simulink model "TorqueSnake"  (R2015b)
settings: Solver=FixedStepAuto  StartTime=0.0  StopTime=tmax  FixedStep=0.01  RelTol=1e-3
values from neighbouring files (symbols this model uses):
  c1 = 0.45    [PreSim.m]
  c2 = 3    [PreSim.m]
  Ms = 1    [PreSim.m]
  N = 3    [PreSim.m]
settings Model: Creator=Christian Dos Santos  LastModifiedBy=Christian Dos Santos

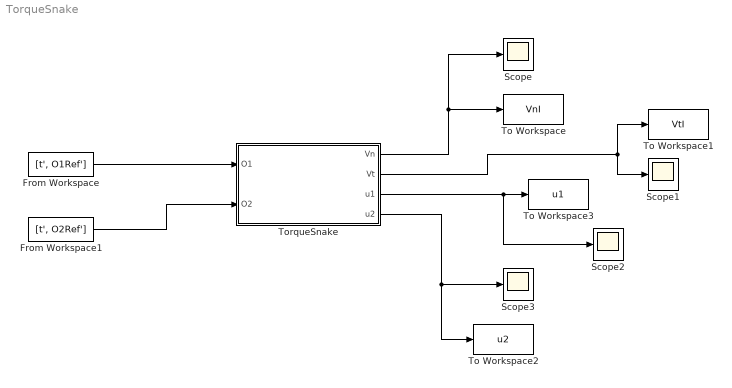
== system TorqueSnake ==
  From Workspace : FromWorkspace  VariableName=[t', O1Ref']
  From Workspace1 : FromWorkspace  VariableName=[t', O2Ref']
  Scope{,1..3} (4 alike) : Scope
  To Workspace : ToWorkspace  VariableName=VnI  SampleTime=-1
  To Workspace1 : ToWorkspace  VariableName=VtI  SampleTime=-1
  To Workspace2 : ToWorkspace  VariableName=u2  SampleTime=-1
  To Workspace3 : ToWorkspace  VariableName=u1  SampleTime=-1
  TorqueSnake : Subsystem
  wires:
  From Workspace/1 -> TorqueSnake/1(O1)
  From Workspace1/1 -> TorqueSnake/2(O2)
  TorqueSnake/1(Vn) -> To Workspace/1, Scope/1
  TorqueSnake/2("Vt ") -> Scope1/1, To Workspace1/1
  TorqueSnake/3(u1) -> To Workspace3/1, Scope2/1
  TorqueSnake/4(u2) -> To Workspace2/1, Scope3/1

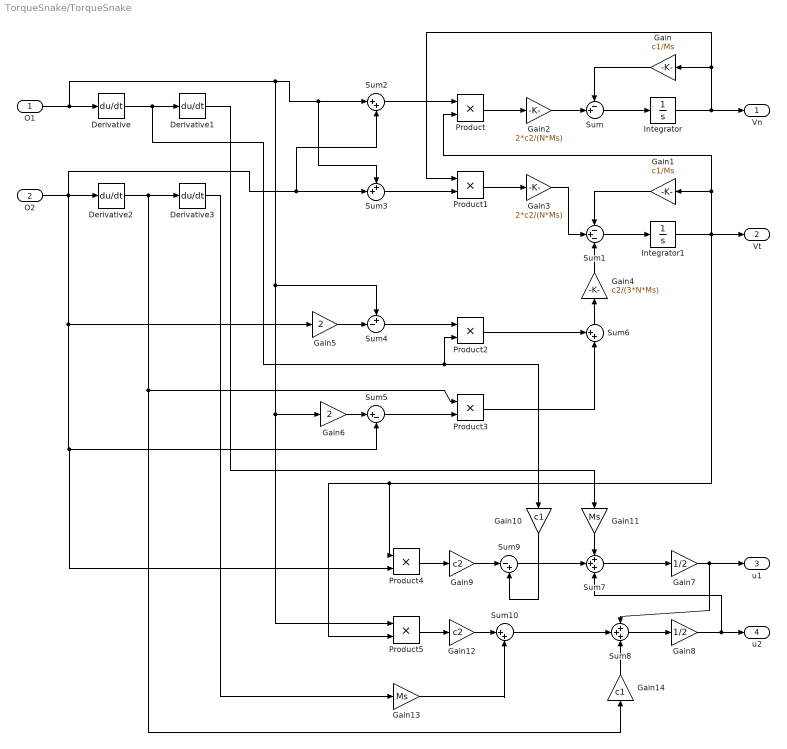
== system TorqueSnake/TorqueSnake ==
  O1 : Inport
  O2 : Inport  Port=2
  Derivative{,1..3} (4 alike) : Derivative
  Gain : Gain  Gain=c1/Ms
  Gain1 : Gain  Gain=c1/Ms
  Gain10 : Gain  Gain=c1
  Gain11 : Gain  Gain=Ms
  Gain12 : Gain  Gain=c2
  Gain13 : Gain  Gain=Ms
  Gain14 : Gain  Gain=c1
  Gain2 : Gain  Gain=2*c2/(N*Ms)
  Gain3 : Gain  Gain=2*c2/(N*Ms)
  Gain4 : Gain  Gain=c2/(3*N*Ms)
  Gain5 : Gain  Gain=2
  Gain6 : Gain  Gain=2
  Gain7 : Gain  Gain=1/2
  Gain8 : Gain  Gain=1/2
  Gain9 : Gain  Gain=c2
  Integrator : Integrator
  Integrator1 : Integrator
  Product{,1..5} (6 alike) : Product
  Sum : Sum  Inputs=-+|
  Sum1 : Sum  Inputs=-+-
  Sum10 : Sum  Inputs=|++
  Sum2 : Sum  Inputs=|++
  Sum3 : Sum  Inputs=++|
  Sum4 : Sum  Inputs=+-|
  Sum5 : Sum  Inputs=|+-
  Sum6 : Sum  Inputs=++|
  Sum7 : Sum  Inputs=+++
  Sum8 : Sum  Inputs=+++
  Sum9 : Sum  Inputs=|-+
  Vn : Outport
  "Vt " : Outport  Port=2
  u1 : Outport  Port=3
  u2 : Outport  Port=4
  wires:
  Integrator/1 -> Gain/1, Product1/1, Vn/1
  Gain/1 -> Sum/1
  Sum/1 -> Integrator/1
  Gain1/1 -> Sum1/1
  Sum1/1 -> Integrator1/1
  O1/1 -> Sum3/1, Sum2/1, Product5/1, Gain6/1, Sum4/1, Derivative/1
  Derivative/1 -> Product2/2, Gain10/1, Derivative1/1
  O2/1 -> Product4/2, Sum5/2, Gain5/1, Sum2/2, Sum3/2, Derivative2/1
  Derivative2/1 -> Product3/1, Gain14/1, Derivative3/1
  Sum3/1 -> Product1/2
  Sum2/1 -> Product/1
  Product/1 -> Gain2/1
  Gain2/1 -> Sum/2
  Product1/1 -> Gain3/1
  Gain3/1 -> Sum1/2
  Product2/1 -> Sum6/1
  Product3/1 -> Sum6/2
  Gain4/1 -> Sum1/3
  Sum6/1 -> Gain4/1
  Sum4/1 -> Product2/1
  Gain5/1 -> Sum4/2
  Sum5/1 -> Product3/2
  Gain6/1 -> Sum5/1
  Gain9/1 -> Sum9/1
  Product4/1 -> Gain9/1
  Gain8/1 -> u2/1, Sum7/3
  Gain10/1 -> Sum9/2
  Sum9/1 -> Sum7/2
  Gain11/1 -> Sum7/1
  Derivative1/1 -> Gain11/1
  Sum7/1 -> Gain7/1
  Gain7/1 -> u1/1, Sum8/1
  Gain12/1 -> Sum10/1
  Product5/1 -> Gain12/1
  Derivative3/1 -> Gain13/1
  Gain13/1 -> Sum10/2
  Sum10/1 -> Sum8/2
  Gain14/1 -> Sum8/3
  Sum8/1 -> Gain8/1
  Integrator1/1 -> Product4/1, Product5/2, Gain1/1, Product/2, "Vt "/1
